simulink model "pil_profiling_am263x"  (R2024b)
settings: Solver=FixedStepAuto  StartTime=0.0  StopTime=5.0  RelTol=1e-3
undefined symbols (not defined in the file): DiscIntNeverNeededParam
libraries: simulink x1, pil_lib x1
settings Model: SILPILSystemUnderTest=refmodels  Creator=a0499511  LastModifiedBy=a0499511
settings OptimizationCC: DefaultParameterBehavior=Inlined  EnhancedBackFolding=on  PassReuseOutputArgsAs=Individual arguments  ZeroExternalMemoryAtStartup=off  ZeroInternalMemoryAtStartup=off  MaxStackSize=64  OptimizeBlockOrder=speed  DifferentSizesBufferReuse=on  OptimizationCustomize=off  EfficientTunableParamExpr=on
settings DebuggingCC: ParameterTunabilityLossMsg=error
settings HardwareCC: ProdBitPerPointer=32  ProdBitPerSizeT=32  ProdBitPerPtrDiffT=32  ProdLargestAtomicInteger=Long  ProdLargestAtomicFloat=Double  ProdWordSize=32  ProdHWDeviceType=ARM Compatible->ARM Cortex
settings SFSimCC: MATLABDynamicMemAlloc=off
settings RTWCC: Description=Embedded Coder  SystemTargetFile=ert.tlc  HardwareBoard=AM263X LP  TemplateMakefile=ert_default_tmf  Toolchain=TI ARM Clang Compiler AM263X | gmake  CreateSILPILBlock=PIL  CodeExecutionProfiling=on  CodeProfilingInstrumentation=coarse
settings CodeAppCC: ForceParamTrailComments=on  IgnoreCustomStorageClasses=off  OperatorAnnotations=on  SimulinkDataObjDesc=on  SFDataObjDesc=on  InsertBlockDesc=on
settings ERTTargetCC: ExtModeTransport=3  ExtModeStaticAlloc=on  ExtModeMexFile=ext_xcp  ExtModeIntrfLevel=Level2 - Open  ERTCustomFileTemplate=AM263x_codertarget_file_process.tlc

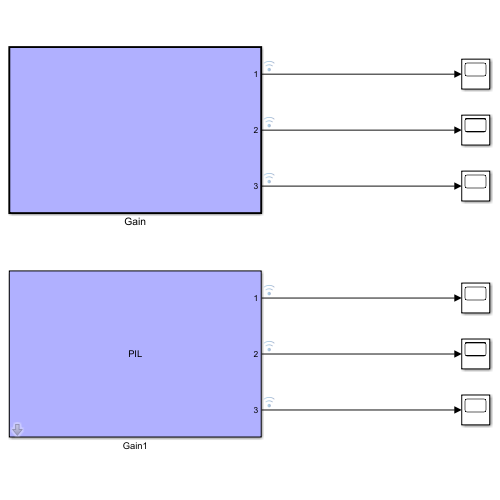
[thumbnail: Simulink's stored preview of the top-level diagram]
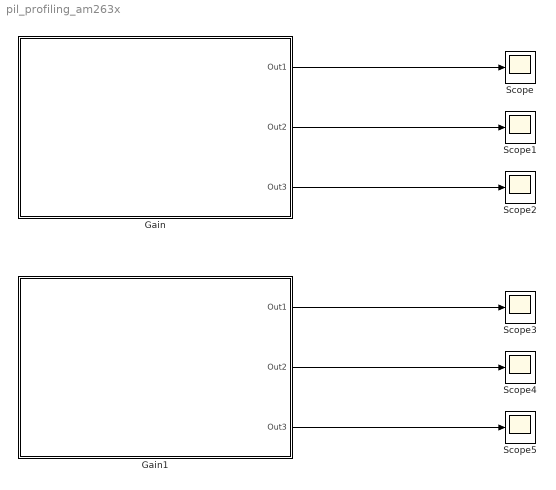
== system pil_profiling_am263x ==
  Gain : Subsystem  TreatAsAtomicUnit=on
  Gain1 : Subsystem  DialogController=pil_create_dialog  LoadFcn=|
      | try
      |    if ~strcmp(rtw.pil.getPILVersion, '24.2 (R2024b)_15')
      |       set_param(gcb, 'DialogController', '');
      |       set_param(gcb, 'DialogControllerArgs', '');
      |    end
      | catch e
      |       set_param(gcb, 'DialogController', '');
      |       set_param(gcb, 'DialogControllerArgs', '');
      | end
      mask help: PIL:pil:XILBlockMaskDesc
      mask Display: disp('PIL');
  Scope{,1..5} (6 alike) : Scope
  wires:
  Gain/1(Out1) -> Scope/1
  Gain/2(Out2) -> Scope1/1
  Gain/3(Out3) -> Scope2/1
  Gain1/1(Out1) -> Scope3/1
  Gain1/3(Out3) -> Scope5/1
  Gain1/2(Out2) -> Scope4/1

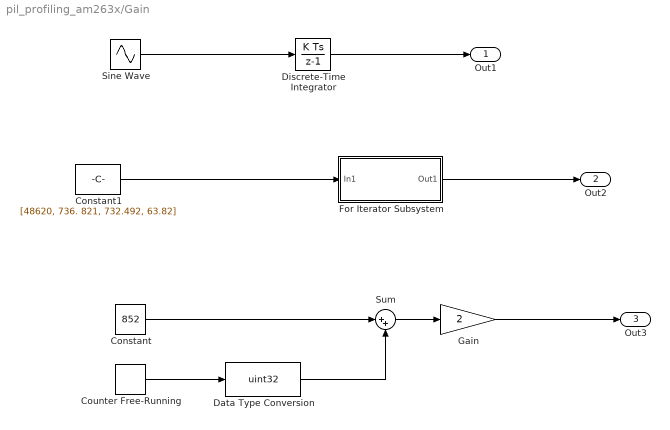
== system pil_profiling_am263x/Gain ==
  Constant : Constant  Value=852  OutDataTypeStr=uint32  SampleTime=200e-6
  Constant1 : Constant  Value=[48620, 736. 821, 732.492, 63.82]  OutDataTypeStr=single  SampleTime=600e-6
  Counter Free-Running : simulink/Sources/Counter Free-Running  NumBits=16  tsamp=-1
  Data Type Conversion : DataTypeConversion  OutDataTypeStr=uint32  SaturateOnIntegerOverflow=off  RndMeth=Floor
  Discrete-Time Integrator : DiscreteIntegrator  gainval=2.0  SampleTime=-1  ICPrevOutput=DiscIntNeverNeededParam  ICPrevScaledInput=DiscIntNeverNeededParam
  For Iterator Subsystem : Subsystem  TreatAsAtomicUnit=on
  Gain : Gain  Gain=2  OutDataTypeStr=uint32
  Sine Wave : Sin  SineType=Sample based  Samples=20  SampleTime=0.001
  Sum : Sum  Inputs=|++
  Out1 : Outport
  Out2 : Outport  Port=2
  Out3 : Outport  Port=3
  wires:
  Discrete-Time Integrator/1 -> Out1/1
  Sine Wave/1 -> Discrete-Time Integrator/1
  For Iterator Subsystem/1(Out1) -> Out2/1
  Constant1/1 -> For Iterator Subsystem/1(In1)
  Gain/1 -> Out3/1
  Sum/1 -> Gain/1
  Counter Free-Running/1 -> Data Type Conversion/1
  Data Type Conversion/1 -> Sum/2
  Constant/1 -> Sum/1

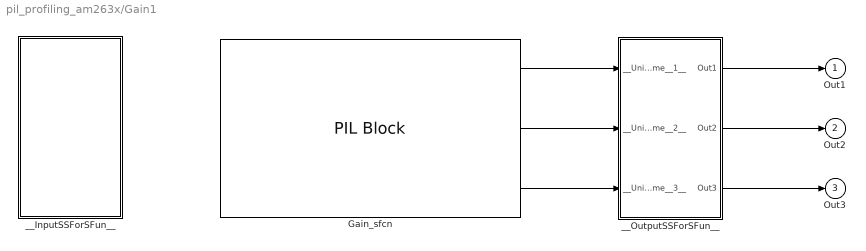
== system pil_profiling_am263x/Gain1 ==
  Gain_sfcn : pil_lib/PIL Block  SimulationMode=PIL  IsTopModelPIL=off  CodeDir=Gain_ert_rtw  AnchorDir=C:\Users\A0499511\development_matlab_simulink\development_matlab_simulink_am26x\examples\pil  ConfigName=AM26X  XrelIsTopModelCode=on  XrelIsReusable=off  XrelDWorkNames={}  XrelDWorkTypes={}  XrelModelArgVals={}  XrelOrderedParamNames={}  XRelNonFiniteStyle=NONFINITE_UNUSED
  __InputSSForSFun__ : Subsystem
  __OutputSSForSFun__ : Subsystem
  Out1 : Outport
  Out2 : Outport  Port=2
  Out3 : Outport  Port=3
  wires:
  Gain_sfcn/1 -> __OutputSSForSFun__/1(__UniqueInportName__1__)
  Gain_sfcn/2 -> __OutputSSForSFun__/2(__UniqueInportName__2__)
  Gain_sfcn/3 -> __OutputSSForSFun__/3(__UniqueInportName__3__)
  __OutputSSForSFun__/1(Out1) -> Out1/1
  __OutputSSForSFun__/2(Out2) -> Out2/1
  __OutputSSForSFun__/3(Out3) -> Out3/1

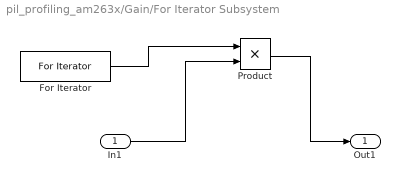
== system pil_profiling_am263x/Gain/For Iterator Subsystem ==
  In1 : Inport
  For Iterator : ForIterator  IterationLimit=250
  Product : Product
  Out1 : Outport
  wires:
  In1/1 -> Product/2
  For Iterator/1 -> Product/1
  Product/1 -> Out1/1

== system pil_profiling_am263x/Gain1/__InputSSForSFun__ ==

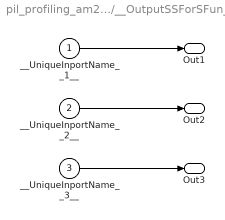
== system pil_profiling_am263x/Gain1/__OutputSSForSFun__ ==
  __UniqueInportName__1__ : Inport
  __UniqueInportName__2__ : Inport  Port=2
  __UniqueInportName__3__ : Inport  Port=3
  Out1 : Outport
  Out2 : Outport  Port=2
  Out3 : Outport  Port=3
  wires:
  __UniqueInportName__1__/1 -> Out1/1
  __UniqueInportName__2__/1 -> Out2/1
  __UniqueInportName__3__/1 -> Out3/1
